simulink model "H_inf_latmod_1_"  (R2025b)
settings: Solver=VariableStepAuto  StartTime=0.0  StopTime=50  RelTol=1e-3
values from neighbouring files (symbols this model uses):
  A_LD = [ ... (first row only)    [Taller1v3.m]    (also in hinf_lat_uav.m; hinf_lat_uav_v2.m)
  B_LD = [ ... (first row only)    [Taller1v3.m]    (also in hinf_lat_uav.m; hinf_lat_uav_v2.m)
  C_LD = [ ... (first row only)    [Taller1v3.m]    (also in hinf_lat_uav.m = C_LD(2:5,:); hinf_lat_uav_v2.m = C_LD(2:5,:))
  D_LD = zeros(4,2)    [Taller1v3.m]    (also in hinf_lat_uav.m; hinf_lat_uav_v2.m)
libraries: simulink x1, robotcorelib x1
settings Model: Creator=57313  LastModifiedBy=Carlo
settings ModelReferenceCC: EnableRefExpFcnMdlSchedulingChecks=on
settings RTWCC: GPUComputeCapability=3.5

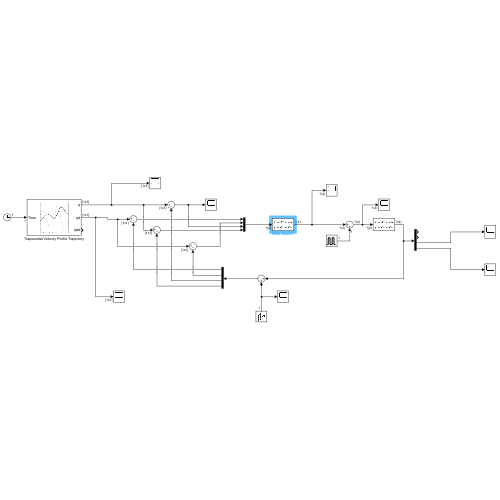
[thumbnail: Simulink's stored preview of the top-level diagram]
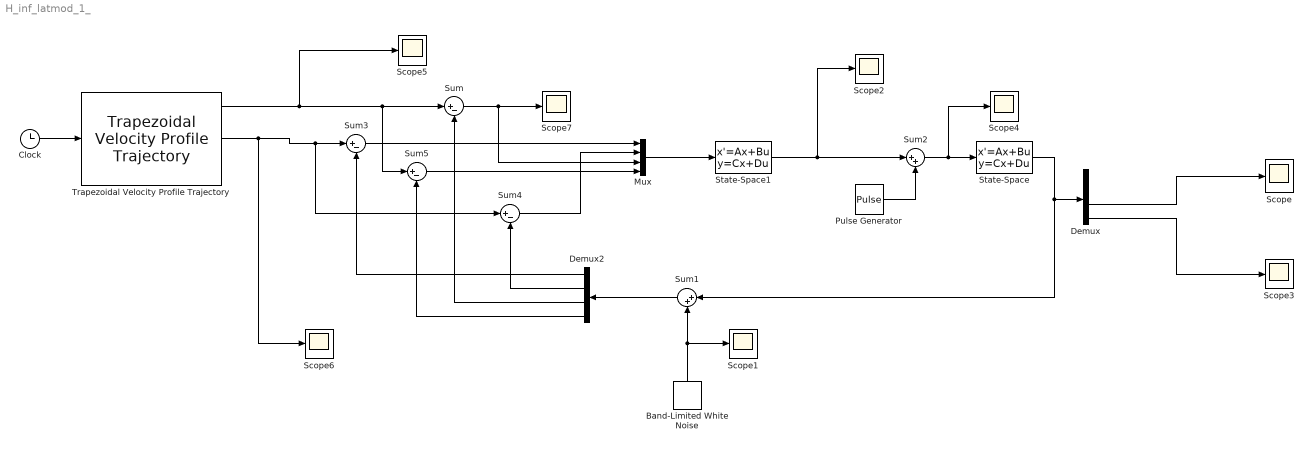
== system H_inf_latmod_1_ ==
  Band-Limited White Noise : simulink/Sources/Band-Limited White Noise  Cov=[0.001]  Ts=0.1  seed=[23341]
  Clock : Clock
  Demux : Demux
  Demux2 : Demux
  Mux : Mux
  Pulse Generator : DiscretePulseGenerator  PulseType=Time based  Amplitude=0  Period=1/6  PulseWidth=50
  Scope{,1..7} (8 alike) : Scope
      Scope settings: ActiveDisplayYMinimum=-0.86532  ActiveDisplayYMaximum=1.63077
      Scope1 settings: ActiveDisplayYMinimum=-0.44423  ActiveDisplayYMaximum=0.3929
      Scope2 settings: ActiveDisplayYMinimum=-0.42893  ActiveDisplayYMaximum=0.4539  DataLoggingVariableName=ScopeData2
      Scope3 settings: ActiveDisplayYMinimum=-0.1749  ActiveDisplayYMaximum=1.18631
      Scope4 settings: ActiveDisplayYMinimum=-13.03819  ActiveDisplayYMaximum=13.17821  DataLoggingVariableName=ScopeData2
      Scope5 settings: ActiveDisplayYMinimum=-0.125  ActiveDisplayYMaximum=1.125
      Scope6 settings: ActiveDisplayYMinimum=-0.1875  ActiveDisplayYMaximum=1.6875  DataLoggingVariableName=ScopeData2
      Scope7 settings: DataLoggingVariableName=ScopeData3
  State-Space : StateSpace  A=A_LD  B=B_LD  C=C_LD  D=D_LD  InitialCondition=[]  ParameterTunability=Unconstrained
  State-Space1 : StateSpace  A=A_LD  B=B_LD  C=C_LD  D=D_LD  InitialCondition=0  ParameterTunability=Unconstrained
  Sum{,3..5} (4 alike) : Sum  Inputs=|+-
  Sum1 : Sum  Inputs=|++
  Sum2 : Sum  Inputs=|++
  Trapezoidal Velocity Profile Trajectory : robotcorelib/Trapezoidal Velocity Profile Trajectory  WaypointSource=Internal  Waypoints=[0 1]  NumParams=1  Parameter1=End Time  Parameter2=End Time  ParameterSource=Internal  PeakVelocity=[ 2; 2 ]  Acceleration=[ 1; 2 ]  EndTime=[ 1 ]  AccelTime=[ 1; 2 ]  SimulateUsing=Interpreted execution
  wires:
  State-Space/1 -> Sum1/1, Demux/1
  State-Space1/1 -> Scope2/1, Sum2/1
  Sum2/1 -> Scope4/1, State-Space/1
  Sum1/1 -> Demux2/1
  Mux/1 -> State-Space1/1
  Sum/1 -> Scope7/1, Mux/3
  Sum3/1 -> Mux/1
  Demux2/1 -> Sum3/2
  Demux2/3 -> Sum/2
  Clock/1 -> Trapezoidal Velocity Profile Trajectory/1
  Band-Limited White Noise/1 -> Sum1/2, Scope1/1
  Trapezoidal Velocity Profile Trajectory/1 -> Scope5/1, Sum5/1, Sum/1
  Trapezoidal Velocity Profile Trajectory/2 -> Scope6/1, Sum4/1, Sum3/1
  Demux2/2 -> Sum4/2
  Sum4/1 -> Mux/2
  Demux2/4 -> Sum5/2
  Sum5/1 -> Mux/4
  Pulse Generator/1 -> Sum2/2
  Demux/3 -> Scope/1
  Demux/4 -> Scope3/1
